simulink subsystem "Gaussian_pulse"  (R2025b)
settings: Solver=VariableStepAuto  StartTime=0.0  StopTime=10.0  RelTol=1e-3
model mask{PeakTime=10, Amplitude=0.15, Sigma=2}
  mask prompts: PeakTime "Peak Time"
settings Model: Creator=klump  LastModifiedBy=klump

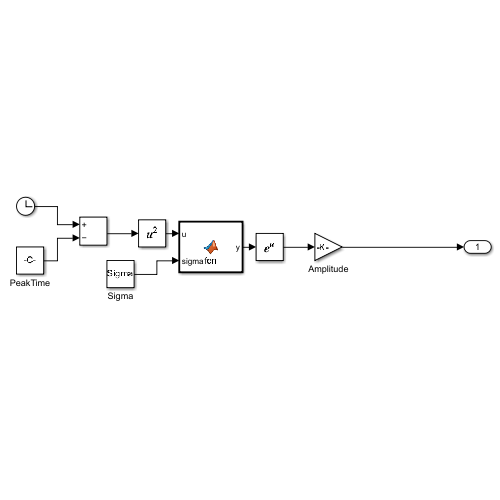
[thumbnail: Simulink's stored preview of the top-level diagram]
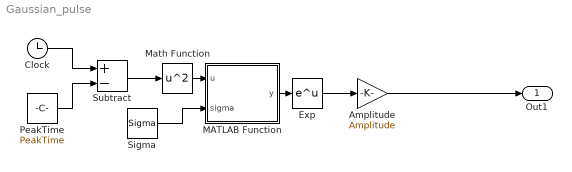
== system Gaussian_pulse ==
  Amplitude : Gain  Gain=Amplitude
  Clock : Clock
  Exp : Math
  MATLAB Function : MATLAB Function  TreatAsAtomicUnit=on
  Math Function : Math  Operator=square
  PeakTime : Constant  Value=PeakTime
  Sigma : Constant  Value=Sigma
  Subtract : Sum  Inputs=+-
  Out1 : Outport
  wires:
  Subtract/1 -> Math Function/1
  Clock/1 -> Subtract/1
  Amplitude/1 -> Out1/1
  PeakTime/1 -> Subtract/2
  Exp/1 -> Amplitude/1
  Math Function/1 -> MATLAB Function/1(u)
  MATLAB Function/1(y) -> Exp/1
  Sigma/1 -> MATLAB Function/2(sigma)

== matlab function Gaussian_pulse/MATLAB Function ==
  data: u input; y output; sigma input
function y = fcn(u,sigma)

y = u*(-1/(2*sigma^2));
